simulink model "Overtaking"  (R2024a)
settings: Solver=FixedStepDiscrete  StartTime=0.0  StopTime=inf  FixedStep=0.001  RelTol=1e-3  EnableMultiTasking=on
undefined symbols (not defined in the file): route1_frenet, route1_waypoint, route2_frenet, route2_waypoint, route3_frenet, route3_waypoint, route4_frenet, route4_waypoint, route5_frenet, route5_waypoint
libraries: CarMaker4SL x49, simulink x1
(part 3 of 4)

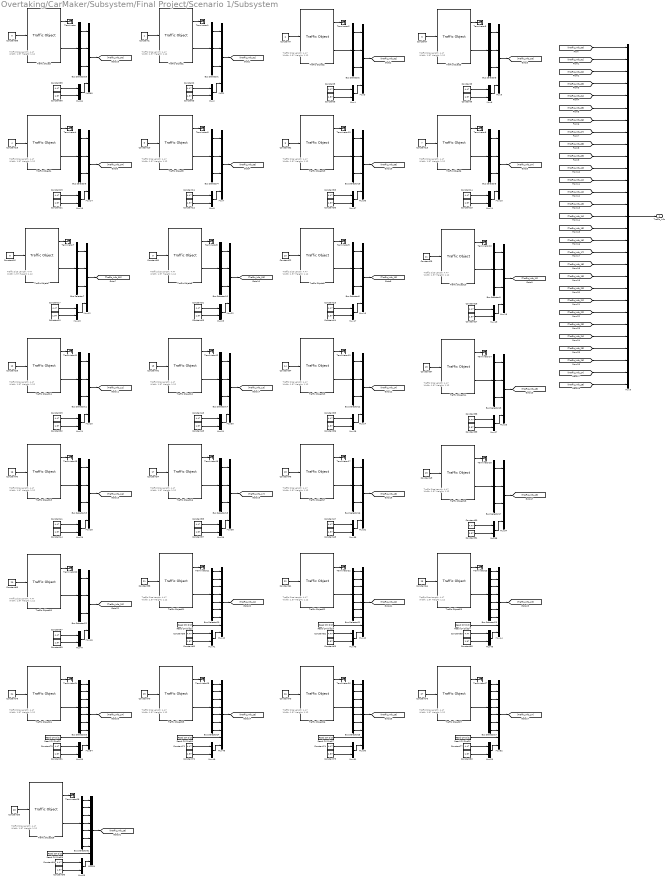
== system Overtaking/CarMaker/Subsystem/Final Project/Scenario 1/Subsystem ==
  note: Traffic Size
      | Length: 4.47
      | Width: 1.97
      | Height: 1.12
  note: Traffic Size
      | Length: 4.47
      | Width: 1.97
      | Height: 1.12
  note: Traffic Size
      | Length: 4.47
      | Width: 1.97
      | Height: 1.12
  note: Traffic Size
      | Length: 4.47
      | Width: 1.97
      | Height: 1.12
  note: Traffic Size
      | Length: 4.47
      | Width: 1.97
      | Height: 1.12
  note: Traffic Size
      | Length: 4.47
      | Width: 1.97
      | Height: 1.12
  note: Traffic Size
      | Length: 4.47
      | Width: 1.97
      | Height: 1.12
  note: Traffic Size
      | Length: 4.47
      | Width: 1.97
      | Height: 1.12
  note: Traffic Size
      | Length: 4.47
      | Width: 1.97
      | Height: 1.12
  note: Traffic Size
      | Length: 4.47
      | Width: 1.97
      | Height: 1.12
  note: Traffic Size
      | Length: 4.47
      | Width: 1.97
      | Height: 1.12
  note: Traffic Size
      | Length: 4.47
      | Width: 1.97
      | Height: 1.12
  note: Traffic Size
      | Length: 4.47
      | Width: 1.97
      | Height: 1.12
  note: Traffic Size
      | Length: 4.47
      | Width: 1.97
      | Height: 1.12
  note: Traffic Size
      | Length: 4.47
      | Width: 1.97
      | Height: 1.12
  note: Traffic Size
      | Length: 4.47
      | Width: 1.97
      | Height: 1.12
  note: Traffic Size
      | Length: 4.47
      | Width: 1.97
      | Height: 1.12
  note: Traffic Size
      | Length: 4.47
      | Width: 1.97
      | Height: 1.12
  note: Traffic Size
      | Length: 4.47
      | Width: 1.97
      | Height: 1.12
  note: Traffic Size
      | Length: 4.47
      | Width: 1.97
      | Height: 1.12
  note: Traffic Size
      | Length: 4.47
      | Width: 1.97
      | Height: 1.12
  note: Traffic Size
      | Length: 4.47
      | Width: 1.97
      | Height: 1.12
  note: Traffic Size
      | Length: 4.47
      | Width: 1.97
      | Height: 1.12
  note: Traffic Size
      | Length: 4.47
      | Width: 1.97
      | Height: 1.12
  note: Traffic Size
      | Length: 4.47
      | Width: 1.97
      | Height: 1.12
  note: Traffic Size
      | Length: 4.47
      | Width: 1.97
      | Height: 1.12
  note: Traffic Size
      | Length: 4.47
      | Width: 1.97
      | Height: 1.12
  note: Traffic Size
      | Length: 4.47
      | Width: 1.97
      | Height: 1.12
  note: Traffic Size
      | Length: 4.47
      | Width: 1.97
      | Height: 1.12
  Bus Selector{1..19,22,29} (21 alike) : BusSelector  OutputSignals=t_0 x,t_0 y,r_zyx z
  Bus Selector{20..21,23..27,31} (8 alike) : BusSelector  OutputSignals=t_0 x,t_0 y,v_0 x,v_0 y,a_0 x,a_0 y,r_zyx z
  Constant1 : Constant
  Constant10 : Constant  Value=5
  Constant{2,5,8,11,14,17,19,23,26,29,31,35,38,41,43,47,50,53,55,59,62,65,67,71,74,77,79,89,94} (29 alike) : Constant  Value=4.47
  Constant{3,6,9,12,15,20..21,24,27,32..33,36,39,44..45,48,51,56..57,60,63,68..69,72,75,80..81,90,96} (29 alike) : Constant  Value=1.97
  Constant13 : Constant  Value=7
  Constant16 : Constant  Value=8
  Constant18 : Constant  Value=4
  Constant22 : Constant  Value=10
  Constant25 : Constant  Value=11
  Constant28 : Constant  Value=12
  Constant30 : Constant  Value=9
  Constant34 : Constant  Value=14
  Constant37 : Constant  Value=15
  Constant4 : Constant  Value=2
  Constant40 : Constant  Value=16
  Constant42 : Constant  Value=13
  Constant46 : Constant  Value=18
  Constant49 : Constant  Value=19
  Constant52 : Constant  Value=6
  Constant54 : Constant  Value=17
  Constant58 : Constant  Value=21
  Constant61 : Constant  Value=22
  Constant64 : Constant  Value=23
  Constant66 : Constant  Value=20
  Constant7 : Constant  Value=3
  Constant70 : Constant  Value=25
  Constant73 : Constant  Value=26
  Constant76 : Constant  Value=27
  Constant78 : Constant  Value=24
  Constant88 : Constant  Value=0
  Constant93 : Constant  Value=28
  Mux{1,3,5,7,10,12,14,16,18,20,22,24,26,28,30,32,34,36,38,46,60} (21 alike) : Mux
  Mux{2,4,6,8,11,13,15,17,19,21,23,25,27,29,31,33,35,37,39,41,43,45,47,49,51,53,55,61,65} (29 alike) : Mux  Inputs=2
  Mux{40,42,44,48,50,52,54,64} (8 alike) : Mux  Inputs=9
  Mux9 : Mux  Inputs=29
  Read CM Dict22 : CarMaker4SL/Read CM Dict  xname=Traffic.T21.rzv  xsync=off  xstime=Inherited
  Read CM Dict23 : CarMaker4SL/Read CM Dict  xname=Traffic.T22.rzv  xsync=off  xstime=Inherited
  Read CM Dict24 : CarMaker4SL/Read CM Dict  xname=Traffic.T23.rzv  xsync=off  xstime=Inherited
  Read CM Dict25 : CarMaker4SL/Read CM Dict  xname=Traffic.T24.rzv  xsync=off  xstime=Inherited
  Read CM Dict26 : CarMaker4SL/Read CM Dict  xname=Traffic.T25.rzv  xsync=off  xstime=Inherited
  Read CM Dict27 : CarMaker4SL/Read CM Dict  xname=Traffic.T26.rzv  xsync=off  xstime=Inherited
  Read CM Dict28 : CarMaker4SL/Read CM Dict  xname=Traffic.T27.rzv  xsync=off  xstime=Inherited
  Read CM Dict29 : CarMaker4SL/Read CM Dict  xname=Traffic.T28.rzv  xsync=off  xstime=Inherited
  Terminator{,1..28} (29 alike) : Terminator
  Traffic Object : CarMaker4SL/Traffic Object  xname=T00  ximode=Traffic Id  xstime=Inherited
      settings: SourceProductName=CarMaker4SL
  Traffic Object1 : CarMaker4SL/Traffic Object  xname=T01  ximode=Traffic Id  xstime=Inherited
      settings: SourceProductName=CarMaker4SL
  Traffic Object10 : CarMaker4SL/Traffic Object  xname=T11  ximode=Traffic Id  xstime=Inherited
      settings: SourceProductName=CarMaker4SL
  Traffic Object11 : CarMaker4SL/Traffic Object  xname=T12  ximode=Traffic Id  xstime=Inherited
      settings: SourceProductName=CarMaker4SL
  Traffic Object12 : CarMaker4SL/Traffic Object  xname=T13  ximode=Traffic Id  xstime=Inherited
      settings: SourceProductName=CarMaker4SL
  Traffic Object13 : CarMaker4SL/Traffic Object  xname=T14  ximode=Traffic Id  xstime=Inherited
      settings: SourceProductName=CarMaker4SL
  Traffic Object14 : CarMaker4SL/Traffic Object  xname=T15  ximode=Traffic Id  xstime=Inherited
      settings: SourceProductName=CarMaker4SL
  Traffic Object15 : CarMaker4SL/Traffic Object  xname=T16  ximode=Traffic Id  xstime=Inherited
      settings: SourceProductName=CarMaker4SL
  Traffic Object16 : CarMaker4SL/Traffic Object  xname=T17  ximode=Traffic Id  xstime=Inherited
      settings: SourceProductName=CarMaker4SL
  Traffic Object17 : CarMaker4SL/Traffic Object  xname=T18  ximode=Traffic Id  xstime=Inherited
      settings: SourceProductName=CarMaker4SL
  Traffic Object18 : CarMaker4SL/Traffic Object  xname=T19  ximode=Traffic Id  xstime=Inherited
      settings: SourceProductName=CarMaker4SL
  Traffic Object19 : CarMaker4SL/Traffic Object  xname=T06  ximode=Traffic Id  xstime=Inherited
      settings: SourceProductName=CarMaker4SL
  Traffic Object2 : CarMaker4SL/Traffic Object  xname=T02  ximode=Traffic Id  xstime=Inherited
      settings: SourceProductName=CarMaker4SL
  Traffic Object20 : CarMaker4SL/Traffic Object  xname=T20  ximode=Traffic Id  xstime=Inherited
      settings: SourceProductName=CarMaker4SL
  Traffic Object21 : CarMaker4SL/Traffic Object  xname=T21  ximode=Traffic Id  xstime=Inherited
      settings: SourceProductName=CarMaker4SL
  Traffic Object22 : CarMaker4SL/Traffic Object  xname=T22  ximode=Traffic Id  xstime=Inherited
      settings: SourceProductName=CarMaker4SL
  Traffic Object23 : CarMaker4SL/Traffic Object  xname=T23  ximode=Traffic Id  xstime=Inherited
      settings: SourceProductName=CarMaker4SL
  Traffic Object24 : CarMaker4SL/Traffic Object  xname=T24  ximode=Traffic Id  xstime=Inherited
      settings: SourceProductName=CarMaker4SL
  Traffic Object25 : CarMaker4SL/Traffic Object  xname=T25  ximode=Traffic Id  xstime=Inherited
      settings: SourceProductName=CarMaker4SL
  Traffic Object26 : CarMaker4SL/Traffic Object  xname=T26  ximode=Traffic Id  xstime=Inherited
      settings: SourceProductName=CarMaker4SL
  Traffic Object27 : CarMaker4SL/Traffic Object  xname=T27  ximode=Traffic Id  xstime=Inherited
      settings: SourceProductName=CarMaker4SL
  Traffic Object28 : CarMaker4SL/Traffic Object  xname=T28  ximode=Traffic Id  xstime=Inherited
      settings: SourceProductName=CarMaker4SL
  Traffic Object3 : CarMaker4SL/Traffic Object  xname=T03  ximode=Traffic Id  xstime=Inherited
      settings: SourceProductName=CarMaker4SL
  Traffic Object4 : CarMaker4SL/Traffic Object  xname=T04  ximode=Traffic Id  xstime=Inherited
      settings: SourceProductName=CarMaker4SL
  Traffic Object5 : CarMaker4SL/Traffic Object  xname=T05  ximode=Traffic Id  xstime=Inherited
      settings: SourceProductName=CarMaker4SL
  Traffic Object6 : CarMaker4SL/Traffic Object  xname=T07  ximode=Traffic Id  xstime=Inherited
      settings: SourceProductName=CarMaker4SL
  Traffic Object7 : CarMaker4SL/Traffic Object  xname=T08  ximode=Traffic Id  xstime=Inherited
      settings: SourceProductName=CarMaker4SL
  Traffic Object8 : CarMaker4SL/Traffic Object  xname=T09  ximode=Traffic Id  xstime=Inherited
      settings: SourceProductName=CarMaker4SL
  Traffic Object9 : CarMaker4SL/Traffic Object  xname=T10  ximode=Traffic Id  xstime=Inherited
      settings: SourceProductName=CarMaker4SL
  Traffic_Info : Outport
  wires:
  Mux61/1 -> Mux60/4
  Mux41/1 -> Mux40/9
  [Traffic_Info_28] -> Mux9/29
  [Traffic_Info_04] -> Mux9/5
  [Traffic_Info_24] -> Mux9/25
  [Traffic_Info_09] -> Mux9/10
  [Traffic_Info_25] -> Mux9/26
  Read CM Dict23/1 -> Mux42/8
  Mux40/1 -> [Traffic_Info_21]
  Read CM Dict24/1 -> Mux44/8
  Constant58/1 -> Traffic Object21/1
  Bus Selector21/7 -> Mux42/7  "<r_zyx z>"
  Bus Selector20/6 -> Mux40/6  "<a_0 y>"
  Bus Selector23/4 -> Mux44/4  "<v_0 y>"
  Traffic Object23/2 -> Bus Selector23/1
  Bus Selector23/7 -> Mux44/7  "<r_zyx z>"
  Bus Selector21/2 -> Mux42/2  "<t_0 y>"
  Constant63/1 -> Mux43/2
  Constant68/1 -> Mux45/2
  Bus Selector25/1 -> Mux50/1  "<t_0 x>"
  Bus Selector10/2 -> Mux22/2  "<t_0 y>"
  Mux28/1 -> [Traffic_Info_16]
  Constant43/1 -> Mux31/1
  Constant81/1 -> Mux55/2
  Bus Selector29/3 -> Mux60/3  "<r_zyx z>"
  Bus Selector16/2 -> Mux32/2  "<t_0 y>"
  Read CM Dict25/1 -> Mux54/8
  Constant21/1 -> Mux15/2
  Bus Selector11/2 -> Mux20/2  "<t_0 y>"
  Mux19/1 -> Mux18/4
  Bus Selector20/7 -> Mux40/7  "<r_zyx z>"
  Bus Selector18/1 -> Mux38/1  "<t_0 x>"
  Traffic Object21/2 -> Bus Selector20/1
  Traffic Object16/2 -> Bus Selector18/1
  Mux31/1 -> Mux30/4
  Mux33/1 -> Mux32/4
  Constant54/1 -> Traffic Object16/1
  [Traffic_Info_11] -> Mux9/12
  Bus Selector31/1 -> Mux64/1  "<t_0 x>"
  Mux26/1 -> [Traffic_Info_15]
  Bus Selector15/1 -> Mux28/1  "<t_0 x>"
  Traffic Object26/2 -> Bus Selector25/1
  Mux35/1 -> Mux34/4
  Constant55/1 -> Mux39/1
  Constant37/1 -> Traffic Object14/1
  Bus Selector17/2 -> Mux34/2  "<t_0 y>"
  Constant11/1 -> Mux8/1
  Constant46/1 -> Traffic Object17/1
  Traffic Object18/2 -> Bus Selector17/1
  Constant50/1 -> Mux35/1
  Bus Selector17/3 -> Mux34/3  "<r_zyx z>"
  Traffic Object/1 -> Terminator/1
  Traffic Object18/1 -> Terminator18/1
  Constant57/1 -> Mux39/2
  Traffic Object17/2 -> Bus Selector16/1
  [Traffic_Info_06] -> Mux9/7
  Traffic Object15/1 -> Terminator15/1
  Mux44/1 -> [Traffic_Info_23]
  Constant14/1 -> Mux11/1
  Bus Selector23/1 -> Mux44/1  "<t_0 x>"
  Bus Selector27/5 -> Mux52/5  "<a_0 x>"
  Constant88/1 -> Traffic Object/1
  Bus Selector26/4 -> Mux54/4  "<v_0 y>"
  Bus Selector24/6 -> Mux48/6  "<a_0 y>"
  Bus Selector25/6 -> Mux50/6  "<a_0 y>"
  Mux48/1 -> [Traffic_Info_25]
  Bus Selector26/5 -> Mux54/5  "<a_0 x>"
  Bus Selector29/1 -> Mux60/1  "<t_0 x>"
  Bus Selector26/1 -> Mux54/1  "<t_0 x>"
  Traffic Object27/1 -> Terminator27/1
  Traffic Object27/2 -> Bus Selector27/1
  Constant52/1 -> Traffic Object19/1
  Bus Selector26/7 -> Mux54/7  "<r_zyx z>"
  Traffic Object13/2 -> Bus Selector12/1
  Constant48/1 -> Mux33/2
  Constant47/1 -> Mux33/1
  Mux23/1 -> Mux22/4
  Traffic Object17/1 -> Terminator17/1
  Bus Selector19/3 -> Mux36/3  "<r_zyx z>"
  Bus Selector23/6 -> Mux44/6  "<a_0 y>"
  Traffic Object20/1 -> Terminator20/1
  Traffic Object1/2 -> Bus Selector1/1
  Constant66/1 -> Traffic Object20/1
  Traffic Object12/1 -> Terminator12/1
  Constant76/1 -> Traffic Object27/1
  Traffic Object10/1 -> Terminator10/1
  Bus Selector22/1 -> Mux46/1  "<t_0 x>"
  [Traffic_Info_20] -> Mux9/21
  Constant75/1 -> Mux51/2
  Mux47/1 -> Mux46/4
  Bus Selector26/3 -> Mux54/3  "<v_0 x>"
  Mux29/1 -> Mux28/4
  [Traffic_Info_13] -> Mux9/14
  Bus Selector6/2 -> Mux14/2  "<t_0 y>"
  Constant18/1 -> Traffic Object4/1
  Constant12/1 -> Mux8/2
  Constant1/1 -> Traffic Object1/1
  Bus Selector6/1 -> Mux14/1  "<t_0 x>"
  Bus Selector3/1 -> Mux5/1  "<t_0 x>"
  Mux5/1 -> [Traffic_Info_03]
  Bus Selector31/5 -> Mux64/5  "<a_0 x>"
  Bus Selector3/3 -> Mux5/3  "<r_zyx z>"
  Bus Selector27/6 -> Mux52/6  "<a_0 y>"
  Constant4/1 -> Traffic Object2/1
  Constant6/1 -> Mux4/2
  Bus Selector27/7 -> Mux52/7  "<r_zyx z>"
  Traffic Object2/1 -> Terminator2/1
  Bus Selector2/1 -> Mux3/1  "<t_0 x>"
  Bus Selector21/5 -> Mux42/5  "<a_0 x>"
  [Traffic_Info_14] -> Mux9/15
  Bus Selector20/3 -> Mux40/3  "<v_0 x>"
  Mux2/1 -> Mux1/4
  Bus Selector2/2 -> Mux3/2  "<t_0 y>"
  Constant3/1 -> Mux2/2
  Bus Selector21/4 -> Mux42/4  "<v_0 y>"
  Traffic Object14/2 -> Bus Selector13/1
  Traffic Object28/2 -> Bus Selector31/1
  Mux64/1 -> [Traffic_Info_28]
  Bus Selector31/2 -> Mux64/2  "<t_0 y>"
  Bus Selector23/3 -> Mux44/3  "<v_0 x>"
  Constant74/1 -> Mux51/1
  Read CM Dict27/1 -> Mux50/8
  Traffic Object28/1 -> Terminator28/1
  Traffic Object25/1 -> Terminator25/1
  Traffic Object24/2 -> Bus Selector26/1
  Bus Selector21/1 -> Mux42/1  "<t_0 x>"
  Bus Selector24/1 -> Mux48/1  "<t_0 x>"
  Read CM Dict26/1 -> Mux48/8
  Bus Selector24/3 -> Mux48/3  "<v_0 x>"
  Mux54/1 -> [Traffic_Info_24]
  Constant70/1 -> Traffic Object25/1
  Bus Selector25/7 -> Mux50/7  "<r_zyx z>"
  [Traffic_Info_26] -> Mux9/27
  Mux49/1 -> Mux48/9
  Constant38/1 -> Mux27/1
  Traffic Object23/1 -> Terminator23/1
  Traffic Object14/1 -> Terminator14/1
  Constant45/1 -> Mux31/2
  [Traffic_Info_00] -> Mux9/1
  Traffic Object7/1 -> Terminator7/1
  Constant44/1 -> Mux29/2
  Bus Selector12/3 -> Mux24/3  "<r_zyx z>"
  Bus Selector27/4 -> Mux52/4  "<v_0 y>"
  Mux38/1 -> [Traffic_Info_17]
  [Traffic_Info_01] -> Mux9/2
  Bus Selector23/2 -> Mux44/2  "<t_0 y>"
  Mux50/1 -> [Traffic_Info_26]
  Constant35/1 -> Mux25/1
  Constant28/1 -> Traffic Object11/1
  Constant40/1 -> Traffic Object15/1
  Constant41/1 -> Mux29/1
  Mux53/1 -> Mux52/9
  Mux11/1 -> Mux10/4
  [Traffic_Info_21] -> Mux9/22
  Read CM Dict22/1 -> Mux40/8
  Constant42/1 -> Traffic Object12/1
  Constant34/1 -> Traffic Object13/1
  Constant39/1 -> Mux27/2
  [Traffic_Info_07] -> Mux9/8
  Mux4/1 -> Mux3/4
  Bus Selector10/3 -> Mux22/3  "<r_zyx z>"
  Bus Selector20/2 -> Mux40/2  "<t_0 y>"
  Mux9/1 -> Traffic_Info/1
  Traffic Object26/1 -> Terminator26/1
  Mux3/1 -> [Traffic_Info_02]
  Bus Selector12/2 -> Mux24/2  "<t_0 y>"
  [Traffic_Info_15] -> Mux9/16
  Traffic Object6/2 -> Bus Selector5/1
  Constant8/1 -> Mux6/1
  Constant80/1 -> Mux53/2
  Bus Selector20/5 -> Mux40/5  "<a_0 x>"
  Traffic Object25/2 -> Bus Selector24/1
  [Traffic_Info_03] -> Mux9/4
  Bus Selector9/3 -> Mux18/3  "<r_zyx z>"
  Traffic Object13/1 -> Terminator13/1
  Bus Selector14/3 -> Mux30/3  "<r_zyx z>"
  [Traffic_Info_10] -> Mux9/11
  Mux30/1 -> [Traffic_Info_13]
  Bus Selector15/2 -> Mux28/2  "<t_0 y>"
  Constant26/1 -> Mux19/1
  Constant2/1 -> Mux2/1
  Constant71/1 -> Mux49/1
  Constant25/1 -> Traffic Object10/1
  [Traffic_Info_18] -> Mux9/19
  Mux20/1 -> [Traffic_Info_12]
  Mux51/1 -> Mux50/9
  Constant10/1 -> Traffic Object5/1
  Bus Selector27/1 -> Mux52/1  "<t_0 x>"
  Traffic Object10/2 -> Bus Selector9/1
  Bus Selector31/7 -> Mux64/7  "<r_zyx z>"
  Bus Selector21/3 -> Mux42/3  "<v_0 x>"
  Constant61/1 -> Traffic Object22/1
  Bus Selector11/1 -> Mux20/1  "<t_0 x>"
  [Traffic_Info_05] -> Mux9/6
  [Traffic_Info_27] -> Mux9/28
  Bus Selector31/6 -> Mux64/6  "<a_0 y>"
  Traffic Object3/1 -> Terminator3/1
  Bus Selector4/1 -> Mux7/1  "<t_0 x>"
  Bus Selector11/3 -> Mux20/3  "<r_zyx z>"
  Bus Selector8/3 -> Mux16/3  "<r_zyx z>"
  Constant72/1 -> Mux49/2
  Constant7/1 -> Traffic Object3/1
  Traffic Object11/1 -> Terminator11/1
  Constant65/1 -> Mux45/1
  Mux46/1 -> [Traffic_Info_20]
  Bus Selector21/6 -> Mux42/6  "<a_0 y>"
  Mux21/1 -> Mux20/4
  Mux65/1 -> Mux64/9
  Bus Selector4/2 -> Mux7/2  "<t_0 y>"
  Traffic Object9/2 -> Bus Selector8/1
  [Traffic_Info_12] -> Mux9/13
  Constant64/1 -> Traffic Object23/1
  Constant31/1 -> Mux23/1
  Traffic Object24/1 -> Terminator24/1
  Mux10/1 -> [Traffic_Info_07]
  Traffic Object2/2 -> Bus Selector2/1
  Constant29/1 -> Mux21/1
  Constant23/1 -> Mux17/1
  Bus Selector2/3 -> Mux3/3  "<r_zyx z>"
  Bus Selector24/7 -> Mux48/7  "<r_zyx z>"
  Constant51/1 -> Mux35/2
  Traffic Object/2 -> Bus Selector29/1
  Traffic Object8/2 -> Bus Selector10/1
  Mux13/1 -> Mux12/4
  Bus Selector1/1 -> Mux1/1  "<t_0 x>"
  Read CM Dict28/1 -> Mux52/8
  Bus Selector24/2 -> Mux48/2  "<t_0 y>"
  Mux1/1 -> [Traffic_Info_01]
  Constant89/1 -> Mux61/1
  Bus Selector25/4 -> Mux50/4  "<v_0 y>"
  Bus Selector27/2 -> Mux52/2  "<t_0 y>"
  Traffic Object11/2 -> Bus Selector11/1
  Constant33/1 -> Mux23/2
  Traffic Object8/1 -> Terminator8/1
  Bus Selector7/1 -> Mux12/1  "<t_0 x>"
  Bus Selector10/1 -> Mux22/1  "<t_0 x>"
  Constant22/1 -> Traffic Object9/1
  Traffic Object12/2 -> Bus Selector14/1
  Read CM Dict29/1 -> Mux64/8
  Bus Selector5/1 -> Mux10/1  "<t_0 x>"
  Constant36/1 -> Mux25/2
  Bus Selector23/5 -> Mux44/5  "<a_0 x>"
  Mux25/1 -> Mux24/4
  Bus Selector7/2 -> Mux12/2  "<t_0 y>"
  Mux43/1 -> Mux42/9
  Bus Selector25/3 -> Mux50/3  "<v_0 x>"
  Bus Selector5/3 -> Mux10/3  "<r_zyx z>"
  Traffic Object5/2 -> Bus Selector4/1
  Mux17/1 -> Mux16/4
  Constant13/1 -> Traffic Object6/1
  Constant60/1 -> Mux41/2
  Constant90/1 -> Mux61/2
  Mux55/1 -> Mux54/9
  Mux14/1 -> [Traffic_Info_04]
  [Traffic_Info_23] -> Mux9/24
  Traffic Object6/1 -> Terminator6/1
  Constant62/1 -> Mux43/1
  Constant15/1 -> Mux11/2
  Bus Selector24/5 -> Mux48/5  "<a_0 x>"
  Bus Selector6/3 -> Mux14/3  "<r_zyx z>"
  Mux12/1 -> [Traffic_Info_08]
  Traffic Object5/1 -> Terminator5/1
  [Traffic_Info_08] -> Mux9/9
  Mux7/1 -> [Traffic_Info_05]
  Bus Selector25/2 -> Mux50/2  "<t_0 y>"
  Bus Selector13/3 -> Mux26/3  "<r_zyx z>"
  Bus Selector4/3 -> Mux7/3  "<r_zyx z>"
  Bus Selector16/1 -> Mux32/1  "<t_0 x>"
  Traffic Object7/2 -> Bus Selector7/1
  Constant5/1 -> Mux4/1
  Bus Selector13/1 -> Mux26/1  "<t_0 x>"
  Mux15/1 -> Mux14/4
  Traffic Object4/2 -> Bus Selector6/1
  Mux36/1 -> [Traffic_Info_06]
  [Traffic_Info_16] -> Mux9/17
  Bus Selector18/2 -> Mux38/2  "<t_0 y>"
  Constant24/1 -> Mux17/2
  Constant19/1 -> Mux15/1
  Mux37/1 -> Mux36/4
  Constant16/1 -> Traffic Object7/1
  [Traffic_Info_17] -> Mux9/18
  Traffic Object22/2 -> Bus Selector21/1
  Constant49/1 -> Traffic Object18/1
  Bus Selector18/3 -> Mux38/3  "<r_zyx z>"
  Mux39/1 -> Mux38/4
  Constant53/1 -> Mux37/1
  Mux16/1 -> [Traffic_Info_10]
  Constant94/1 -> Mux65/1
  Constant20/1 -> Mux13/2
  Traffic Object19/1 -> Terminator19/1
  Bus Selector27/3 -> Mux52/3  "<v_0 x>"
  Bus Selector31/3 -> Mux64/3  "<v_0 x>"
  Constant56/1 -> Mux37/2
  Traffic Object3/2 -> Bus Selector3/1
  Traffic Object9/1 -> Terminator9/1
  [Traffic_Info_22] -> Mux9/23
  Bus Selector26/6 -> Mux54/6  "<a_0 y>"
  Bus Selector19/1 -> Mux36/1  "<t_0 x>"
  Bus Selector9/2 -> Mux18/2  "<t_0 y>"
  Traffic Object16/1 -> Terminator16/1
  Bus Selector12/1 -> Mux24/1  "<t_0 x>"
  Bus Selector26/2 -> Mux54/2  "<t_0 y>"
  Bus Selector25/5 -> Mux50/5  "<a_0 x>"
  Constant67/1 -> Mux47/1
  Constant9/1 -> Mux6/2
  Bus Selector16/3 -> Mux32/3  "<r_zyx z>"
  Bus Selector22/2 -> Mux46/2  "<t_0 y>"
  Mux42/1 -> [Traffic_Info_22]
  Mux60/1 -> [Traffic_Info_00]
  Constant17/1 -> Mux13/1
  Constant96/1 -> Mux65/2
  Constant32/1 -> Mux21/2
  Bus Selector14/1 -> Mux30/1  "<t_0 x>"
  Mux8/1 -> Mux7/4
  Bus Selector17/1 -> Mux34/1  "<t_0 x>"
  Bus Selector3/2 -> Mux5/2  "<t_0 y>"
  Traffic Object22/1 -> Terminator22/1
  Bus Selector5/2 -> Mux10/2  "<t_0 y>"
  Bus Selector1/3 -> Mux1/3  "<r_zyx z>"
  Traffic Object4/1 -> Terminator4/1
  Bus Selector15/3 -> Mux28/3  "<r_zyx z>"
  Bus Selector31/4 -> Mux64/4  "<v_0 y>"
  Bus Selector7/3 -> Mux12/3  "<r_zyx z>"
  Constant73/1 -> Traffic Object26/1
  Mux27/1 -> Mux26/4
  Bus Selector8/2 -> Mux16/2  "<t_0 y>"
  Bus Selector1/2 -> Mux1/2  "<t_0 y>"
  Bus Selector22/3 -> Mux46/3  "<r_zyx z>"
  Constant59/1 -> Mux41/1
  [Traffic_Info_02] -> Mux9/3
  Traffic Object15/2 -> Bus Selector15/1
  Mux32/1 -> [Traffic_Info_18]
  Bus Selector9/1 -> Mux18/1  "<t_0 x>"
  Bus Selector13/2 -> Mux26/2  "<t_0 y>"
  Bus Selector19/2 -> Mux36/2  "<t_0 y>"
  Mux18/1 -> [Traffic_Info_11]
  Bus Selector24/4 -> Mux48/4  "<v_0 y>"
  Mux24/1 -> [Traffic_Info_14]
  Constant30/1 -> Traffic Object8/1
  Mux34/1 -> [Traffic_Info_19]
  [Traffic_Info_19] -> Mux9/20
  Bus Selector8/1 -> Mux16/1  "<t_0 x>"
  Bus Selector20/1 -> Mux40/1  "<t_0 x>"
  Mux52/1 -> [Traffic_Info_27]
  Bus Selector14/2 -> Mux30/2  "<t_0 y>"
  Bus Selector29/2 -> Mux60/2  "<t_0 y>"
  Traffic Object21/1 -> Terminator21/1
  Constant77/1 -> Mux53/1
  Constant93/1 -> Traffic Object28/1
  Mux45/1 -> Mux44/9
  Mux22/1 -> [Traffic_Info_09]
  Mux6/1 -> Mux5/4
  Traffic Object19/2 -> Bus Selector19/1
  Constant27/1 -> Mux19/2
  Constant78/1 -> Traffic Object24/1
  Constant69/1 -> Mux47/2
  Constant79/1 -> Mux55/1
  Traffic Object1/1 -> Terminator1/1
  Bus Selector20/4 -> Mux40/4  "<v_0 y>"
  Traffic Object20/2 -> Bus Selector22/1

== system Overtaking/CarMaker/IPG Vehicle/CarAndTrailer/Forces/Suspension Forces/Suspension External Forces Update ==
  Bus Creator21 : BusCreator  Inputs=6
  Bus Creator22 : BusCreator  Inputs=4
  Bus Creator23 : BusCreator  Inputs=4
  From : From  TagVisibility=global
  Ground{32..39} (8 alike) : Ground
  Out1 : Outport
  wires:
  [D] -> Bus Creator21/4
  Ground36/1 -> Bus Creator22/1
  From/1 -> Bus Creator21/1
  [B] -> Bus Creator21/2
  Ground34/1 -> Bus Creator23/3
  Ground32/1 -> Bus Creator23/1
  [C] -> Bus Creator21/3
  Bus Creator23/1 -> Bus Creator21/5
  Ground33/1 -> Bus Creator23/2
  Bus Creator22/1 -> Bus Creator21/6
  Bus Creator21/1 -> Out1/1
  Ground35/1 -> Bus Creator23/4
  Ground39/1 -> Bus Creator22/4
  Ground38/1 -> Bus Creator22/3
  Ground37/1 -> Bus Creator22/2

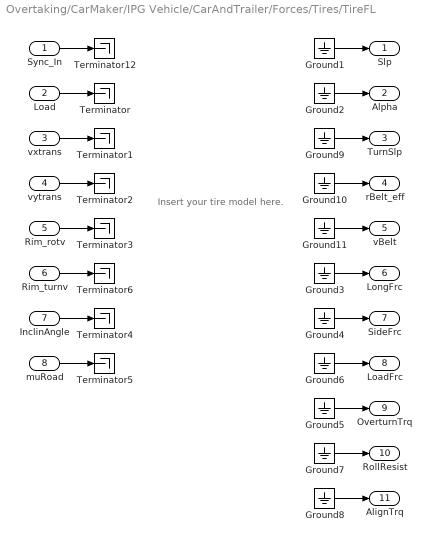
== system Overtaking/CarMaker/IPG Vehicle/CarAndTrailer/Forces/Tires/TireFL ==
  note: Insert your tire model here.
  Sync_In : Inport
  Load : Inport  Port=2
  vxtrans : Inport  Port=3
  vytrans : Inport  Port=4
  Rim_rotv : Inport  Port=5
  Rim_turnv : Inport  Port=6
  InclinAngle : Inport  Port=7
  muRoad : Inport  Port=8
  Ground{1..11} (11 alike) : Ground
  Terminator{,1..6,12} (8 alike) : Terminator
  Slp : Outport  VectorParamsAs1DForOutWhenUnconnected=off
  Alpha : Outport  Port=2  VectorParamsAs1DForOutWhenUnconnected=off
  TurnSlp : Outport  Port=3  VectorParamsAs1DForOutWhenUnconnected=off
  rBelt_eff : Outport  Port=4  VectorParamsAs1DForOutWhenUnconnected=off
  vBelt : Outport  Port=5  VectorParamsAs1DForOutWhenUnconnected=off
  LongFrc : Outport  Port=6  VectorParamsAs1DForOutWhenUnconnected=off
  SideFrc : Outport  Port=7  VectorParamsAs1DForOutWhenUnconnected=off
  LoadFrc : Outport  Port=8  VectorParamsAs1DForOutWhenUnconnected=off
  OverturnTrq : Outport  Port=9  VectorParamsAs1DForOutWhenUnconnected=off
  RollResist : Outport  Port=10  VectorParamsAs1DForOutWhenUnconnected=off
  AlignTrq : Outport  Port=11  VectorParamsAs1DForOutWhenUnconnected=off
  wires:
  Ground11/1 -> vBelt/1
  Ground10/1 -> rBelt_eff/1
  Ground9/1 -> TurnSlp/1
  Rim_turnv/1 -> Terminator6/1
  Sync_In/1 -> Terminator12/1
  Ground2/1 -> Alpha/1
  Ground3/1 -> LongFrc/1
  Ground4/1 -> SideFrc/1
  Ground5/1 -> OverturnTrq/1
  vxtrans/1 -> Terminator1/1
  vytrans/1 -> Terminator2/1
  Rim_rotv/1 -> Terminator3/1
  InclinAngle/1 -> Terminator4/1
  muRoad/1 -> Terminator5/1
  Load/1 -> Terminator/1
  Ground1/1 -> Slp/1
  Ground6/1 -> LoadFrc/1
  Ground7/1 -> RollResist/1
  Ground8/1 -> AlignTrq/1

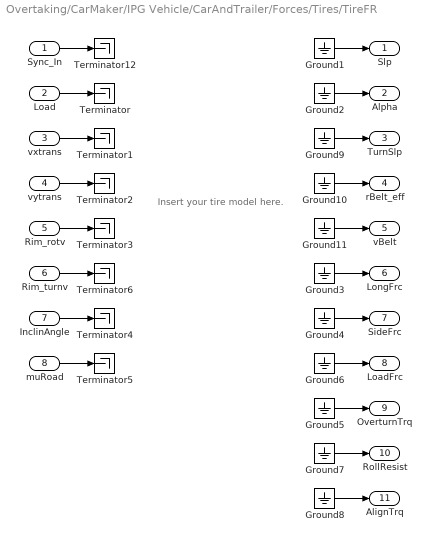
== system Overtaking/CarMaker/IPG Vehicle/CarAndTrailer/Forces/Tires/TireFR ==
  note: Insert your tire model here.
  Sync_In : Inport
  Load : Inport  Port=2
  vxtrans : Inport  Port=3
  vytrans : Inport  Port=4
  Rim_rotv : Inport  Port=5
  Rim_turnv : Inport  Port=6
  InclinAngle : Inport  Port=7
  muRoad : Inport  Port=8
  Ground{1..11} (11 alike) : Ground
  Terminator{,1..6,12} (8 alike) : Terminator
  Slp : Outport  VectorParamsAs1DForOutWhenUnconnected=off
  Alpha : Outport  Port=2  VectorParamsAs1DForOutWhenUnconnected=off
  TurnSlp : Outport  Port=3  VectorParamsAs1DForOutWhenUnconnected=off
  rBelt_eff : Outport  Port=4  VectorParamsAs1DForOutWhenUnconnected=off
  vBelt : Outport  Port=5  VectorParamsAs1DForOutWhenUnconnected=off
  LongFrc : Outport  Port=6  VectorParamsAs1DForOutWhenUnconnected=off
  SideFrc : Outport  Port=7  VectorParamsAs1DForOutWhenUnconnected=off
  LoadFrc : Outport  Port=8  VectorParamsAs1DForOutWhenUnconnected=off
  OverturnTrq : Outport  Port=9  VectorParamsAs1DForOutWhenUnconnected=off
  RollResist : Outport  Port=10  VectorParamsAs1DForOutWhenUnconnected=off
  AlignTrq : Outport  Port=11  VectorParamsAs1DForOutWhenUnconnected=off
  wires:
  Ground11/1 -> vBelt/1
  Ground10/1 -> rBelt_eff/1
  Ground9/1 -> TurnSlp/1
  Rim_turnv/1 -> Terminator6/1
  Sync_In/1 -> Terminator12/1
  Ground2/1 -> Alpha/1
  Ground3/1 -> LongFrc/1
  Ground4/1 -> SideFrc/1
  Ground5/1 -> OverturnTrq/1
  vxtrans/1 -> Terminator1/1
  vytrans/1 -> Terminator2/1
  Rim_rotv/1 -> Terminator3/1
  InclinAngle/1 -> Terminator4/1
  muRoad/1 -> Terminator5/1
  Load/1 -> Terminator/1
  Ground1/1 -> Slp/1
  Ground6/1 -> LoadFrc/1
  Ground7/1 -> RollResist/1
  Ground8/1 -> AlignTrq/1

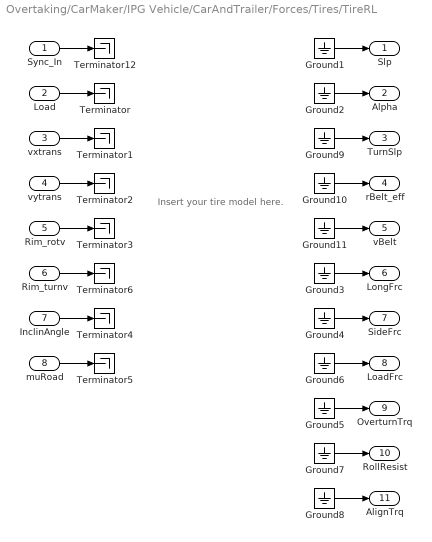
== system Overtaking/CarMaker/IPG Vehicle/CarAndTrailer/Forces/Tires/TireRL ==
  note: Insert your tire model here.
  Sync_In : Inport
  Load : Inport  Port=2
  vxtrans : Inport  Port=3
  vytrans : Inport  Port=4
  Rim_rotv : Inport  Port=5
  Rim_turnv : Inport  Port=6
  InclinAngle : Inport  Port=7
  muRoad : Inport  Port=8
  Ground{1..11} (11 alike) : Ground
  Terminator{,1..6,12} (8 alike) : Terminator
  Slp : Outport  VectorParamsAs1DForOutWhenUnconnected=off
  Alpha : Outport  Port=2  VectorParamsAs1DForOutWhenUnconnected=off
  TurnSlp : Outport  Port=3  VectorParamsAs1DForOutWhenUnconnected=off
  rBelt_eff : Outport  Port=4  VectorParamsAs1DForOutWhenUnconnected=off
  vBelt : Outport  Port=5  VectorParamsAs1DForOutWhenUnconnected=off
  LongFrc : Outport  Port=6  VectorParamsAs1DForOutWhenUnconnected=off
  SideFrc : Outport  Port=7  VectorParamsAs1DForOutWhenUnconnected=off
  LoadFrc : Outport  Port=8  VectorParamsAs1DForOutWhenUnconnected=off
  OverturnTrq : Outport  Port=9  VectorParamsAs1DForOutWhenUnconnected=off
  RollResist : Outport  Port=10  VectorParamsAs1DForOutWhenUnconnected=off
  AlignTrq : Outport  Port=11  VectorParamsAs1DForOutWhenUnconnected=off
  wires:
  Ground11/1 -> vBelt/1
  Ground10/1 -> rBelt_eff/1
  Ground9/1 -> TurnSlp/1
  Rim_turnv/1 -> Terminator6/1
  Sync_In/1 -> Terminator12/1
  Ground2/1 -> Alpha/1
  Ground3/1 -> LongFrc/1
  Ground4/1 -> SideFrc/1
  Ground5/1 -> OverturnTrq/1
  vxtrans/1 -> Terminator1/1
  vytrans/1 -> Terminator2/1
  Rim_rotv/1 -> Terminator3/1
  InclinAngle/1 -> Terminator4/1
  muRoad/1 -> Terminator5/1
  Load/1 -> Terminator/1
  Ground1/1 -> Slp/1
  Ground6/1 -> LoadFrc/1
  Ground7/1 -> RollResist/1
  Ground8/1 -> AlignTrq/1

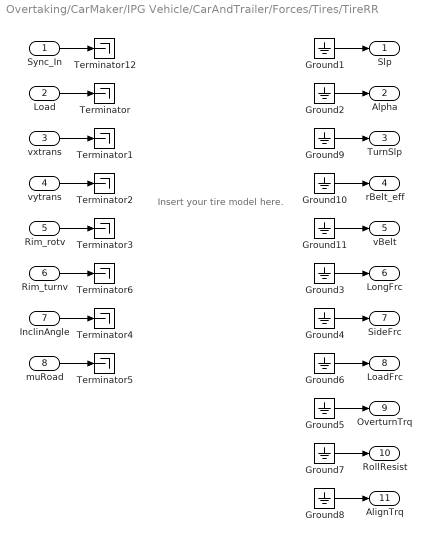
== system Overtaking/CarMaker/IPG Vehicle/CarAndTrailer/Forces/Tires/TireRR ==
  note: Insert your tire model here.
  Sync_In : Inport
  Load : Inport  Port=2
  vxtrans : Inport  Port=3
  vytrans : Inport  Port=4
  Rim_rotv : Inport  Port=5
  Rim_turnv : Inport  Port=6
  InclinAngle : Inport  Port=7
  muRoad : Inport  Port=8
  Ground{1..11} (11 alike) : Ground
  Terminator{,1..6,12} (8 alike) : Terminator
  Slp : Outport  VectorParamsAs1DForOutWhenUnconnected=off
  Alpha : Outport  Port=2  VectorParamsAs1DForOutWhenUnconnected=off
  TurnSlp : Outport  Port=3  VectorParamsAs1DForOutWhenUnconnected=off
  rBelt_eff : Outport  Port=4  VectorParamsAs1DForOutWhenUnconnected=off
  vBelt : Outport  Port=5  VectorParamsAs1DForOutWhenUnconnected=off
  LongFrc : Outport  Port=6  VectorParamsAs1DForOutWhenUnconnected=off
  SideFrc : Outport  Port=7  VectorParamsAs1DForOutWhenUnconnected=off
  LoadFrc : Outport  Port=8  VectorParamsAs1DForOutWhenUnconnected=off
  OverturnTrq : Outport  Port=9  VectorParamsAs1DForOutWhenUnconnected=off
  RollResist : Outport  Port=10  VectorParamsAs1DForOutWhenUnconnected=off
  AlignTrq : Outport  Port=11  VectorParamsAs1DForOutWhenUnconnected=off
  wires:
  Ground11/1 -> vBelt/1
  Ground10/1 -> rBelt_eff/1
  Ground9/1 -> TurnSlp/1
  Rim_turnv/1 -> Terminator6/1
  Sync_In/1 -> Terminator12/1
  Ground2/1 -> Alpha/1
  Ground3/1 -> LongFrc/1
  Ground4/1 -> SideFrc/1
  Ground5/1 -> OverturnTrq/1
  vxtrans/1 -> Terminator1/1
  vytrans/1 -> Terminator2/1
  Rim_rotv/1 -> Terminator3/1
  InclinAngle/1 -> Terminator4/1
  muRoad/1 -> Terminator5/1
  Load/1 -> Terminator/1
  Ground1/1 -> Slp/1
  Ground6/1 -> LoadFrc/1
  Ground7/1 -> RollResist/1
  Ground8/1 -> AlignTrq/1

== matlab function Overtaking/CarMaker/Subsystem/Final Project/Scenario 1/MATLAB Function1 ==
  data: lane_id input; route_waypoint output; route_frenet output; route1_waypoint input; route1_frenet input; route2_waypoint input; route2_frenet input; route3_waypoint input; route3_frenet input; route4_waypoint input; route4_frenet input; route5_waypoint input; route5_frenet input
function [route_waypoint, route_frenet] = select_lane(lane_id, route1_waypoint, ...
    route1_frenet, route2_waypoint, route2_frenet, route3_waypoint, route3_frenet, ...
    route4_waypoint, route4_frenet, route5_waypoint, route5_frenet)

    [route_waypoint, route_frenet] = select_lane_func(lane_id, route1_waypoint, ...
    route1_frenet, route2_waypoint, route2_frenet, route3_waypoint, route3_frenet, ...
    route4_waypoint, route4_frenet, route5_waypoint, route5_frenet);
end

== matlab function Overtaking/CarMaker/Subsystem/Final Project/Scenario 1/MATLAB Function4 1 ==
  settings: sampleTime=0.1
  data: waypoints input; local_wp output; vehicle_position input; heading input
function local_wp = global_to_local_waypoints(waypoints, vehicle_position, heading)

    waypoints_x = waypoints(:,1);
    waypoints_y = waypoints(:,2);
    num_points = length(waypoints_x);

    local_wp = zeros(num_points, 2);
    x_ego = vehicle_position(1);
    y_ego = vehicle_position(2);
    
    for i = 1:num_points
        dx = waypoints_x(i) - x_ego;
        dy = waypoints_y(i) - y_ego;

        local_x = dx * cos(-heading) - dy * sin(-heading);
        local_y = dx * sin(-heading) + dy * cos(-heading);

        local_wp(i, :) = [local_x, local_y];
    end    
end

== matlab function Overtaking/CarMaker/Subsystem/Final Project/Scenario 1/Waypoint_Follower2 ==
  settings: sampleTime=0.1
  data: local_waypoints input; optimal_local input; steering_angle output; state input; change_dist input; target_idx output
% local tracking
function [steering_angle, target_idx] = waypoint_follower(local_waypoints, optimal_local, state, change_dist)

    WHEEL_BASE = 2.9;
    lookahead_dist = 6.0;
    
    % sigmoid lookahead_dist change
    if(change_dist > 1.8) 
        lookahead_dist = (10 / (1 + exp(-0.4 * change_dist))) + 5;
    end
    % 
    % % final state -> parking area entry
    if(state == 7)
        lookahead_dist = 2.5;
    end

    target_idx = -1;
    final_ld = 0;
    if(state == 0)
        for i = 1:size(optimal_local, 1)
            dist = norm(optimal_local(i, :));
            if dist > lookahead_dist && optimal_local(i, 1) > 0
                target_idx = i;
                final_ld = dist;
                break;
            end
        end

        if target_idx == -1
            steering_angle = 0;
            return;
        end

        target_point = optimal_local(target_idx, :);
        alpha = atan2(target_point(2), target_point(1));
        alpha = wrapToPi(alpha);
    else 
        for i = 1:size(local_waypoints, 1)
            dist = norm(local_waypoints(i, :));
            if dist > lookahead_dist && local_waypoints(i, 1) > 0
                target_idx = i;
                final_ld = dist;
                break;
            end
        end
    
        if target_idx == -1
            steering_angle = 0;
            return;
        end
    
        target_point = local_waypoints(target_idx, :);
        alpha = atan2(target_point(2), target_point(1));
        alpha = wrapToPi(alpha);
    end
    % for i = 1:size(local_waypoints, 1)
    %     dist = norm(local_waypoints(i, :));
    %     if dist > lookahead_dist && local_waypoints(i, 1) > 0
    %         target_idx = i;
    %         final_ld = dist;
    %         break;
    %     end
    % end
    % 
    % if target_idx == -1
    %     steering_angle = 0;
    %     return;
    % end
    % 
    % target_point = local_waypoints(target_idx, :);
    % alpha = atan2(target_point(2), target_point(1));
    % alpha = wrapToPi(alpha);

    final_ld = min(max(final_ld, 2.0), 20.0); 

    steering_angle = atan2(2 * WHEEL_BASE * sin(alpha), final_ld);
end


% % global tracking
% function [steering_angle, start_idx] = pure_pursuit(waypoints, vehicle_position, head)
% 
%     persistent last_target_idx;
%     if isempty(last_target_idx)
%         last_target_idx = 1; % 초기값 설정
%     end
% 
%     WHEEL_BASE = 2.7;
% 
%     waypoints_x = waypoints(:,1);
%     waypoints_y = waypoints(:,2);
%     % num_points = length(waypoints_x);
%     num_points = 300;
% 
%     local_waypoints = zeros(num_points, 2);
%     x_ego = vehicle_position(1);
%     y_ego = vehicle_position(2);
% 
%     for i = 1:num_points
%         dx = waypoints_x(i) - x_ego;
%         dy = waypoints_y(i) - y_ego;
% 
%         local_x = dx * cos(-head) - dy * sin(-head);
%         local_y = dx * sin(-head) + dy * cos(-head);
% 
%         local_waypoints(i, :) = [local_x, local_y];
%     end    
% 
%     lookahead_dist = 5.0;
% 
%     distances_to_waypoints = sqrt((waypoints_x - x_ego).^2 + (waypoints_y - y_ego).^2);
%     [~, closest_idx] = min(distances_to_waypoints);
% 
%     start_idx = max(last_target_idx, closest_idx);
% 
%     target_idx = -1;
%     final_ld = 0;
%     for i = start_idx:num_points
%         dist = norm(local_waypoints(i, :));
%         if dist > lookahead_dist && local_waypoints(i, 1) > 0
%             target_idx = i;
%             final_ld = dist;
%             break;
%         end
%     end
% 
%     if target_idx == -1
%         for i = 1:start_idx-1
%             dist = norm(local_waypoints(i, :));
%             if dist > lookahead_dist && local_waypoints(i, 1) > 0
%                 target_idx = i;
%                 final_ld = dist;
%                 break;
%             end
%         end
%     end
% 
%     if target_idx == -1
%         steering_angle = 0;
%         return;
%     end
% 
%     target_point = local_waypoints(target_idx, :);
%     alpha = atan2(target_point(2), target_point(1));
%     alpha = wrapToPi(alpha);
% 
%     final_ld = min(max(final_ld, 2.0), 20.0);
% 
%     steering_angle = atan2(2 * WHEEL_BASE * sin(alpha), final_ld);
% 
%     last_target_idx = target_idx;
% end

== matlab function Overtaking/CarMaker/Subsystem/Final Project/Scenario 1/MATLAB Function2 ==
  data: candidate_paths_cartesian input; valid_idx output; obs_xy input
function valid_idx = apply_constraint_to_candidate_func(candidate_paths_cartesian, obs_xy)

    valid_idx = apply_constraint_to_candidate_func(candidate_paths_cartesian, obs_xy);

    % for i = 1:length(valid_idx)
    %     idx = valid_idx(i);
    %     valid_paths = candidate_paths_cartesian(:, :, idx);  % [N x 2] 크기
    % end
end

== matlab function Overtaking/CarMaker/Subsystem/Final Project/Scenario 1/MATLAB Function12 ==
  settings: sampleTime=0.1
  data: ego_velocity input; desired_ax output; target_velocity input
function desired_ax = longitudinal_speed_pid_controller_(ego_velocity, target_velocity)
    persistent Kp Kd prev_error dt

    % 초기화 (한 번만 실행)
    if isempty(prev_error)
        Kp = 1.0;     % 비례 이득
        Kd = 0.0;     % 미분 이득
        dt = 0.001;    % 제어 주기 (초)
        prev_error = 0;
    end

    % 오차 계산
    error = target_velocity - ego_velocity;
    d_error = (error - prev_error) / dt;

    % PD 제어 계산
    desired_ax = Kp * error + Kd * d_error;

    % 상태 업데이트
    prev_error = error;
end

== matlab function Overtaking/CarMaker/Subsystem/Final Project/Scenario 1/MATLAB Function4 ==
  data: u input; Ego_s output; Ego_ds output; Ego_dds output; Ego_d output; Ego_dd output; Ego_ddd output
function [Ego_s, Ego_ds, Ego_dds, Ego_d, Ego_dd, Ego_ddd] = fcn(u)
    
    Ego_s = u(1);
    Ego_ds = u(2);
    Ego_dds = u(3);
    Ego_d = u(4);
    Ego_dd = u(5);
    Ego_ddd = u(6);

end

== matlab function Overtaking/CarMaker/Subsystem/Final Project/Scenario 1/MATLAB Function5 ==
  data: route input; candidate_paths output; route1_frenet input; route3_frenet input; ego_s input; ego_d input
function candidate_paths = generate_candidate_paths(route, route1_frenet, route3_frenet, ego_s, ego_d)
    global_s = route(:,1);
    global_d = route(:,2);
    
    % lane_width를 고정값으로 가정
    lane_width = 19;         % 차선 폭: 3.5
    num_lateral_paths = 5;  % 반드시 홀수 (중앙값이 0이 되도록)
    
    % d
    % 왼쪽이 양수
    % 오른쪽이 음수
    
    % 중앙값이 0이 되도록 등간격 리스트 생성
    half_range = lane_width/2;
    step = 2 * half_range / (num_lateral_paths - 1);
    deviation_list = -half_range : step : half_range;
    
    if isequal(route, route1_frenet)
        % if ego_d > 0
        %     deviation_list(deviation_list > 0) = 0; % 차량이 왼쪽 차선의 바깥쪽에 붙은 경우 중앙~오른쪽만 허용
        % end 
        deviation_list(deviation_list > 0) = 0;
    end
    
    if isequal(route, route3_frenet)
        % if ego_d < 0
        %     deviation_list(deviation_list < 0) = 0;  % 차량이 오른쪽 차선의 바깥쪽에 붙은 경우 차선은 중앙~왼쪽만 허용
        % end
        deviation_list(deviation_list < 0) = 0;
    end
    
    % 경로 설정 파라미터
    lookahead_index  = 5;          % lookahead_index
    num_points = 20;
    
    candidate_paths = generate_candidate_paths_func( ...
        global_s, global_d, ego_s, ego_d, deviation_list, lookahead_index , num_points);
end

== matlab function Overtaking/CarMaker/Subsystem/Final Project/Scenario 1/MATLAB Function7 ==
  data: candidate_paths input; path_costs output; opt_d input; target_speed input; dt input
% function [path_costs, s_path, d_path] = calculate_path_costs(candidate_paths, opt_d, target_speed, dt)
%     outside_cost = 2e6;
%     path_costs = calculate_path_costs_func(candidate_paths, opt_d, target_speed, dt);    % 후보 경로마다 cost 계산
%     path_costs(3) = path_costs(3) + outside_cost;
%     [s_path, d_path] = select_lowest_cost_path(candidate_paths, path_costs);        % minimum cost인 경로 (s, d) 추출
% 
%     % d_path_len : 20
%     % s_path_len : 20
% end

function path_costs = calculate_path_costs(candidate_paths, opt_d, target_speed, dt)
    path_costs = calculate_path_costs_func(candidate_paths, opt_d, target_speed, dt);    % 후보 경로마다 cost 계산

end

== matlab function Overtaking/CarMaker/Subsystem/Final Project/Scenario 1/MATLAB Function8 ==
  data: optimal_path input; cartesian_path output; route_waypoints input; num_points output
function [cartesian_path, num_points] = convert_all_frenet_to_cartesian(optimal_path, route_waypoints)

    [cartesian_path, num_points] = convert_all_frenet_to_cartesian_func(optimal_path, route_waypoints);
end

== matlab function Overtaking/CarMaker/Subsystem/Final Project/Scenario 1/MATLAB Function6 ==
  data: valid_idx input; optimal_path output; candidates_cost input; candidate_paths_cartesian input; num_points output; best_idx output; candidates_cost output
function [optimal_path, num_points, best_idx, candidates_cost] = collision_check(valid_idx, candidates_cost, candidate_paths_cartesian)

    [optimal_path, num_points, best_idx, candidates_cost] = collision_check_func(valid_idx, candidates_cost, candidate_paths_cartesian);
end

== matlab function Overtaking/CarMaker/Subsystem/Final Project/Scenario 1/Waypoint_Loader ==
  data: lane_1 input; local_waypoints output; lane_2 input; lane_3 input; lane_4 input; lane_5 input; state output; vehicle_pos input; heading input; closest_waypoint_idx output; lane_num output; speed output; change_dist output
function [local_waypoints, state, closest_waypoint_idx, lane_num, speed, change_dist] = waypoint_loader(lane_1, lane_2, lane_3, lane_4, lane_5, vehicle_pos, heading)
    
    lane_5 = [lane_5; 2.38, -36.18; 3.17, -36.47; 4, -36.6; 4.5, -36.6; 5.0, -36.6; 5.5, -36.6];

    persistent lap_count;
    if isempty(lap_count)
        lap_count = 1;
    end
    persistent entry_5;
    if isempty(entry_5)
        entry_5 = 1;
    end

    lane = lane_2; 
    state = 0;
    lane_num = 0;
    speed = 0;
    change_dist = 0;

    distances = sqrt((lane(:,1) - vehicle_pos(1)).^2 + (lane(:,2) - vehicle_pos(2)).^2);
    [~, closest_waypoint_idx] = min(distances);

    if lap_count == 1
        if closest_waypoint_idx < 18
            lane = lane_2;
            lane_num = 2;
            speed = 50;
            state = 0;
        elseif closest_waypoint_idx < 55
            lane = lane_1;
            lane_num = 1;
            speed = 50;
            state = 0;
        elseif closest_waypoint_idx < 87
            lane = lane_2;
            lane_num = 2;
            speed = 50;
            state = 0;
        elseif closest_waypoint_idx < 125
            lane = lane_1;
            lane_num = 1;
            speed = 50;
            state = 0;
        elseif closest_waypoint_idx < 180
            lane = lane_2;
            lane_num = 2;
            state = 0;
            speed = 50;
        elseif closest_waypoint_idx < 187
            lane = lane_1;
            lane_num = 1;
            state = 1;
            speed = 50;
        elseif closest_waypoint_idx < 190
            lane = lane_2;
            lane_num = 2;
            state = 2;
            speed = 50;
        elseif closest_waypoint_idx < 224
            lane = lane_3;
            lane_num = 3;
            state = 3;
            speed = 50;
            lap_count = lap_count + 1;
        else
            lane = lane_2;
            lane_num = 2;
            speed = 50;
        end


    else
        lane = lane_3;
        if closest_waypoint_idx < 9
            lane = lane_3;
            lane_num = 50;
            state = 5;
            speed = 50;
        elseif closest_waypoint_idx < 22
            lane = lane_4;
            lane_num = 80;
            speed = 30;
            entry_5 = entry_5 + 1;
            state = 6;
        elseif entry_5 > 1
            lane = lane_5;
            lane_num = 200;
            state = 7;
            speed = 10;
        else 
            lane = lane_3;
            lane_num = 100; 
            state = 4;
            speed = 50;
        end
    end

    % closest_waypoint 
    distances = sqrt((lane(:,1) - vehicle_pos(1)).^2 + (lane(:,2) - vehicle_pos(2)).^2);
    [~, closest_waypoint_idx] = min(distances);
    start_idx = closest_waypoint_idx;
    
    % lane_change diff dist
    dx_c = lane(closest_waypoint_idx, 1) - vehicle_pos(1);
    dy_c = lane(closest_waypoint_idx, 2) - vehicle_pos(2);
    change_dist = sqrt(dx_c^2 + dy_c^2);

    % 10 waypoint select
    end_idx = min(start_idx + 9, size(lane, 1));
    selected_waypoints = lane(start_idx:end_idx, :);

    % local transform
    local_waypoints = zeros(size(selected_waypoints));
    for i = 1:size(selected_waypoints, 1)
        dx = selected_waypoints(i, 1) - vehicle_pos(1);
        dy = selected_waypoints(i, 2) - vehicle_pos(2);

        local_x = dx * cos(-heading) - dy * sin(-heading);
        local_y = dx * sin(-heading) + dy * cos(-heading);

        local_waypoints(i, :) = [local_x, local_y];
    end
end

% function [local_waypoints, state, closest_waypoint_idx, lane_num] = waypoint_loader(lane_1, lane_2, lane_3, lane_4, lane_5, vehicle_pos, heading)
% 
%     persistent lap_count current_lane_num;
%     if isempty(lap_count)
%         lap_count = 1;
%     end
% 
%     if isempty(current_lane_num)
%         current_lane_num = 2;
%     end
% 
%     lane_list = {lane_1, lane_2, lane_3, lane_4, lane_5};
% 
%     current_lane = lane_list{current_lane_num};
%     distances = sqrt((current_lane(:,1) - vehicle_pos(1)).^2 + (current_lane(:,2) - vehicle_pos(2)).^2);
%     [~, closest_waypoint_idx] = min(distances);
% 
%     if lap_count == 1
%         if  closest_waypoint_idx > 200
%             current_lane_num = 1; 
%         elseif closest_waypoint_idx > 210
%             current_lane_num = 2; 
%         elseif  closest_waypoint_idx > 223
%             current_lane_num = 3;
%             lap_count = lap_count + 1;
%         else 
%             current_lane_num = 2;
%         end
%     else
%         % --- Lap 2 이상 로직 ---
%         if current_lane_num == 3 && closest_waypoint_idx > 10
%             current_lane_num = 4;
%         elseif current_lane_num == 4 && closest_waypoint_idx > 15
%             current_lane_num = 5;
%         end
%     end
% 
%     % 최종 lane 정보
%     lane = lane_list{current_lane_num};
%     lane_num = current_lane_num;
% 
%     % 최신 lane에 대해 closest waypoint 재계산
%     distances = sqrt((lane(:,1) - vehicle_pos(1)).^2 + (lane(:,2) - vehicle_pos(2)).^2);
%     [~, closest_waypoint_idx] = min(distances);
% 
% 
%     start_idx = closest_waypoint_idx;
%     end_idx = min(start_idx + 9, size(lane, 1));
%     selected_waypoints = lane(start_idx:end_idx, :);
% 
%     local_waypoints = zeros(size(selected_waypoints));
%     for i = 1:size(selected_waypoints, 1)
%         dx = selected_waypoints(i, 1) - vehicle_pos(1);
%         dy = selected_waypoints(i, 2) - vehicle_pos(2);
% 
%         local_x = dx * cos(-heading) - dy * sin(-heading);
%         local_y = dx * sin(-heading) + dy * cos(-heading);
% 
%         local_waypoints(i, :) = [local_x, local_y];
%     end
% 
%     state = 0; % 필요에 따라 갱신
% 
% end

== matlab function Overtaking/CarMaker/Subsystem/Final Project/Scenario 1/MATLAB Function10 ==
  data: traffic_info input; obs_xy output
function obs_xy = mux_traffics_xy(traffic_info)

    obs_xy = mux_traffics_xy_func(traffic_info);
end

== matlab function Overtaking/CarMaker/Subsystem/Final Project/Scenario 1/MATLAB Function3 ==
  settings: sampleTime=0.1
  data: ego_velocity input; desired_ax output; target_velocity input
function desired_ax = longitudinal_speed_pid_controller_(ego_velocity, target_velocity)
    persistent Kp Kd prev_error dt

    % 초기화 (한 번만 실행)
    if isempty(prev_error)
        Kp = 1.0;     % 비례 이득
        Kd = 0.0;     % 미분 이득
        dt = 0.001;    % 제어 주기 (초)
        prev_error = 0;
    end

    % 오차 계산
    error = target_velocity - ego_velocity;
    d_error = (error - prev_error) / dt;

    % PD 제어 계산
    desired_ax = Kp * error + Kd * d_error;

    % 상태 업데이트
    prev_error = error;
end

== matlab function Overtaking/CarMaker/Subsystem/Final Project/Scenario 1/MATLAB Function4 2 ==
  settings: sampleTime=0.1
  data: waypoints input; local_wp output; vehicle_position input; heading input
function local_wp = global_to_local_waypoints(waypoints, vehicle_position, heading)

    waypoints_x = waypoints(:,1);
    waypoints_y = waypoints(:,2);
    num_points = length(waypoints_x);

    local_wp = zeros(num_points, 2);
    x_ego = vehicle_position(1);
    y_ego = vehicle_position(2);
    
    for i = 1:num_points
        dx = waypoints_x(i) - x_ego;
        dy = waypoints_y(i) - y_ego;

        local_x = dx * cos(-heading) - dy * sin(-heading);
        local_y = dx * sin(-heading) + dy * cos(-heading);

        local_wp(i, :) = [local_x, local_y];
    end    
end

== matlab function Overtaking/CarMaker/Subsystem/Final Project/Scenario 1/MATLAB Function ==
  data: waypoints input; EgoFrenet output; interval input; egoState input
function EgoFrenet = convertPathToFrenet(waypoints, interval, egoState)

    EgoFrenet = convertPathToFrenet(waypoints, interval, egoState);
end
